simulink model "sistema_4"  (R2018a)
settings: Solver=VariableStepAuto  StartTime=0.0  StopTime=15  MaxStep=1e-3  RelTol=1e-3
settings Model: Creator=carma  LastModifiedBy=carma

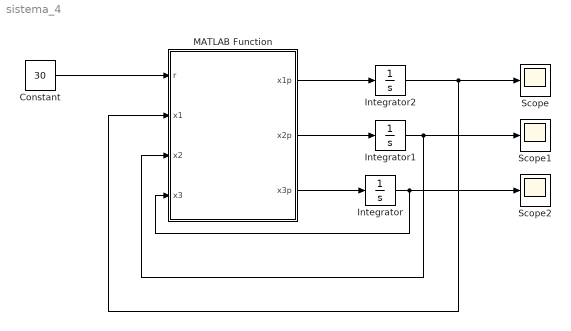
== system sistema_4 ==
  Constant : Constant  Value=30
  Integrator : Integrator
  Integrator1 : Integrator
  Integrator2 : Integrator
  MATLAB Function : MATLAB Function  TreatAsAtomicUnit=on
  Scope : Scope
  Scope1 : Scope
  Scope2 : Scope
  wires:
  MATLAB Function/3(x3p) -> Integrator/1
  MATLAB Function/2(x2p) -> Integrator1/1
  MATLAB Function/1(x1p) -> Integrator2/1
  Integrator/1 -> Scope2/1, MATLAB Function/4(x3)
  Integrator1/1 -> Scope1/1, MATLAB Function/3(x2)
  Integrator2/1 -> Scope/1, MATLAB Function/2(x1)
  Constant/1 -> MATLAB Function/1(r)

== matlab function sistema_4/MATLAB Function ==
  data: r input; x1p output; x1 input; x2 input; x3 input; x2p output; x3p output
function [x1p,x2p,x3p] = fcn(r,x1,x2,x3)
%Parametros

Ra=1000;
La=1e-3;
Ks=0.5;
Ka=10;
kb=0.25;
ki=0.25;
M=0.2; %0.5
k=1;
b=3;

%X(1)=i X(2)=x  X(3)=xp
e=Ka*(r-x2)*Ks;
F=ki*x1;
fem=kb*x3;
x1p=(e-Ra*x1-fem)/La;
x2p=x3;
x3p=(F-b*x3-k*x2)/M;
% xp=[x1p x2p x3p]';
